simulink model "diagrama2"  (R2024b)
settings: Solver=VariableStepAuto  StartTime=0.0  StopTime=10.0  RelTol=1e-3
settings Model: Creator=Iustin  LastModifiedBy=Iustin
settings RTWCC: GPUComputeCapability=3.5

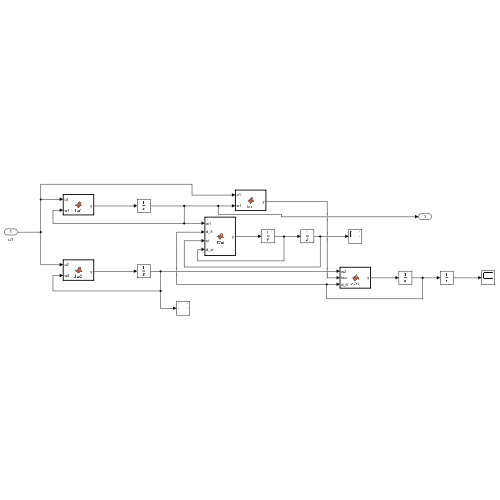
[thumbnail: Simulink's stored preview of the top-level diagram]
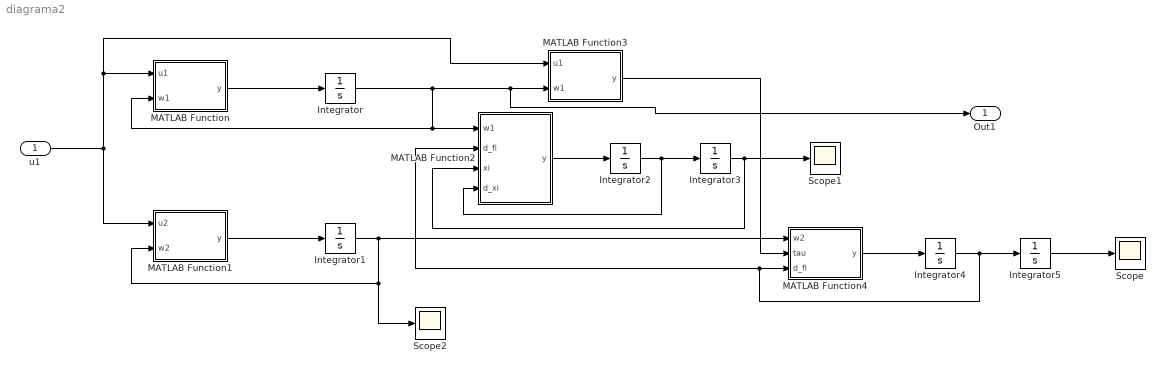
== system diagrama2 ==
  u1 : Inport
  Integrator{,1..5} (6 alike) : Integrator  InitialCondition=1
  MATLAB Function : MATLAB Function  TreatAsAtomicUnit=on
  MATLAB Function1 : MATLAB Function  TreatAsAtomicUnit=on
  MATLAB Function2 : MATLAB Function  TreatAsAtomicUnit=on
  MATLAB Function3 : MATLAB Function  TreatAsAtomicUnit=on
  MATLAB Function4 : MATLAB Function  TreatAsAtomicUnit=on
  Scope : Scope
  Scope1 : Scope
  Scope2 : Scope
  Out1 : Outport
  wires:
  u1/1 -> MATLAB Function1/1(u2), MATLAB Function/1(u1), MATLAB Function3/1(u1)
  MATLAB Function1/1(y) -> Integrator1/1
  MATLAB Function/1(y) -> Integrator/1
  Integrator1/1 -> Scope2/1, MATLAB Function1/2(w2), MATLAB Function4/1(w2)
  Integrator/1 -> MATLAB Function/2(w1), MATLAB Function2/1(w1), MATLAB Function3/2(w1), Out1/1
  Integrator4/1 -> MATLAB Function4/3(d_fi), MATLAB Function2/2(d_fi), Integrator5/1
  MATLAB Function4/1(y) -> Integrator4/1
  Integrator5/1 -> Scope/1
  MATLAB Function3/1(y) -> MATLAB Function4/2(tau)
  Integrator3/1 -> MATLAB Function2/3(xi), Scope1/1
  MATLAB Function2/1(y) -> Integrator2/1
  Integrator2/1 -> MATLAB Function2/4(d_xi), Integrator3/1

== matlab function diagrama2/MATLAB Function1 ==
  data: u2 input; y output; w2 input
function y = dw2(u2, w2)

I2 = 2;
Ki2 = 1000;
R2 = 1000;
K2 = 0.21;
Kb2 = 1;
B2 = 0.001;
C2 = 0.001;
Bp2 = 1;
Dp2 = 1;

y = (1/I2)*((Ki2/R2)*(K2*u2-Kb2*w2)-(B2*w2+C2*sign(w2))-(Bp2*w2+Dp2*w2*w2));

== matlab function diagrama2/MATLAB Function ==
  data: u1 input; y output; w1 input
function y = dw1(u1,w1)

I1 = 1.25;
Ki1 = 1000;
R1 = 1000;
K1 = 0.53;
Kb1 = 1;
B1 = 0.001;
C1 = 0.001;
Bp1 = 1;
Dp1 =1;


y = (1/I1)*((Ki1/R1)*(K1*u1-Kb1*w1)-(B1*w1+C1*sign(w1))-(Bp1*w1+Dp1*w1*w1));

== matlab function diagrama2/MATLAB Function2 ==
  data: w1 input; y output; d_fi input; xi input; d_xi input
function y = d2xi(w1,d_fi,xi,d_xi)

I_elevatie = 0.00437;
Kw1 = 1;
B_elevatie = 0.001 * 1.8;
C_elevatie = 0;
m = 0.0117;
g = 10;
l = 0.33;
K_gyro = 0.015;

y = (1/I_elevatie)*(Kw1*w1*w1-(B_elevatie*d_xi+C_elevatie*sign(d_xi))-m*g*l*sin(xi)-K_gyro*cos(xi)*w1*w1*d_fi-(m*l/2)*sin(2*xi)*d_fi*d_fi);

== matlab function diagrama2/MATLAB Function3 ==
  data: u1 input; y output; w1 input
function y = tau(u1,w1)

Ki1 = 1000;
R1 = 1000;
K1 = 0.53;
Kb1 = 1;
B1 = 0.001;
C1 = 0.001;

y = (Ki1/R1)*(K1*u1-Kb1*w1)-(B1*w1+C1*sign(w1));

== matlab function diagrama2/MATLAB Function4 ==
  data: w2 input; y output; tau input; d_fi input
function y = d2fi(w2,tau,d_fi)

I_azimut = 0.00414;
Kw2 = 1;
B_azimut = 0.001 * 8.69;
C_azimut = 0;

a = Kw2 * (w2 ^ 2);
b = B_azimut * d_fi + C_azimut * sign(d_fi);

y = (1/I_azimut)*(Kw2*w2*w2-tau-(B_azimut*d_fi+C_azimut*sign(d_fi)));
